simulink model "ssbdemo"  (Simulink 8.3)
settings: Solver=FixedStepDiscrete  SolverMode=SingleTasking  StartTime=0.0  StopTime=99999999  RelTol=1e-3  AbsTol=1e-6
libraries: dspsrcs4 x2, dspxfrm3 x1, dspmisc x1
settings Model: Creator=The MathWorks Inc.  CovMetricSettings=d  ExtModeTrigMode=oneshot  ExtModeArmWhenConnect=off
settings DataIOCC: LimitDataPoints=off  SaveOutput=off  SaveTime=off
settings OptimizationCC: BlockReduction=off  BooleanDataType=off  ExpressionDepthLimit=2147483647  RollThreshold=2  InitFltsAndDblsToZero=on
settings DebuggingCC: SaveWithParameterizedLinksMsg=none  SignalResolutionControl=TryResolveAllWithWarning  SolverPrmCheckMsg=none  MultiTaskDSMMsg=warning  MultiTaskCondExecSysMsg=none  IntegerOverflowMsg=none  FcnCallInpInsideContextMsg=UseLocalSettings  StrictBusMsg=None
settings HardwareCC: TargetUnknown=on
settings RTWCC: IncludeERTFirstTime=on
settings GRTTargetCC: TargetFcnLib=ansi_tfl_tmw.mat

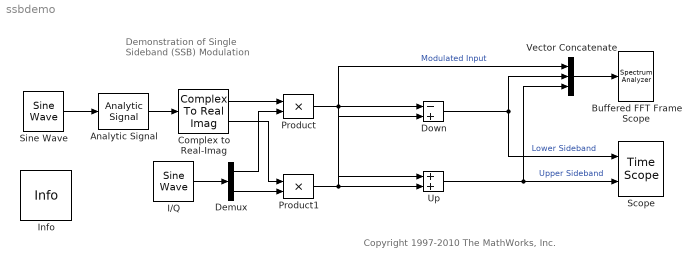
== system ssbdemo ==
  note: Demonstration of
      | Single Sideband (SSB)
      | Modulation
  note: Copyright 1997-2010 The MathWorks, Inc.
  Analytic Signal : dspxfrm3/Analytic Signal  N=100
  Buffered FFT Frame Scope : SpectrumAnalyzer  ScopeSpecification=DataTag1
  Complex to Real-Imag : ComplexToRealImag
  Demux : Demux  Outputs=2
  Down : Sum  Inputs=-+  SaturateOnIntegerOverflow=on  InputSameDT=on  OutDataTypeStr=Inherit: Same as first input
  I/Q : dspsrcs4/Sine Wave  Amplitude=1  Frequency=2  Phase=[0 pi/2]  SampleMode=Discrete  OutComplex=Real  CompMethod=Trigonometric fcn  TableSize=Speed  SampleTime=0.1  SamplesPerFrame=1  ResetState=Restart at time zero  dataType=double  wordLen=16  udDataType=sfix(16)  fracBitsMode=Best precision  numFracBits=15  OutDataTypeStr=double  LastOutDataTypeStr=double
  Info : dspmisc/Info  SystemSampleTime=-1
  Product : Product  SaturateOnIntegerOverflow=on  RndMeth=Zero  InputSameDT=on  OutDataTypeStr=Inherit: Same as first input
  Product1 : Product  SaturateOnIntegerOverflow=on  RndMeth=Zero  InputSameDT=on  OutDataTypeStr=Inherit: Same as first input
  Scope : TimeScope  NumInputPorts=2  DefaultConfigurationName=spbscopes.TimeScopeBlockCfg  ScopeSpecification=DataTag2
  Sine Wave : dspsrcs4/Sine Wave  Amplitude=1  Frequency=0.5  Phase=0  SampleMode=Discrete  OutComplex=Real  CompMethod=Trigonometric fcn  TableSize=Speed  SampleTime=0.1  SamplesPerFrame=1  ResetState=Restart at time zero  dataType=double  wordLen=16  udDataType=sfix(16)  fracBitsMode=Best precision  numFracBits=15  OutDataTypeStr=double  LastOutDataTypeStr=double
  Up : Sum  SaturateOnIntegerOverflow=on  InputSameDT=on  OutDataTypeStr=Inherit: Same as first input
  Vector Concatenate : Concatenate  NumInputs=3  Mode=Multidimensional array  ConcatenateDimension=2
  wires:
  Sine Wave/1 -> Analytic Signal/1
  Analytic Signal/1 -> Complex to Real-Imag/1
  Product/1 -> Down/1, Up/1, Vector Concatenate/1  "Modulated Input"
  Product1/1 -> Up/2, Down/2
  Complex to Real-Imag/2 -> Product1/1
  Demux/2 -> Product1/2
  Complex to Real-Imag/1 -> Product/1
  Demux/1 -> Product/2
  Down/1 -> Scope/1, Vector Concatenate/2  "Lower Sideband"
  Up/1 -> Scope/2, Vector Concatenate/3  "Upper Sideband"
  I/Q/1 -> Demux/1
  Vector Concatenate/1 -> Buffered FFT Frame Scope/1
